simulink library "DAEMOT_Lib"  (R2019b)
settings: Solver=ode45  StartTime=0.0  StopTime=10.0  FixedStep=0.1  RelTol=1e-3
undefined symbols (not defined in the file or in its folder): Controller, CP, Ctrl, Ctrl_Fcn, Elec1, f, F2, Fluid, lag1, Mission, Moody, PropellerProp, rev_comms_sink
libraries: $bdroot x200, instrumentlib x21, simulink x5, dspsigops x2
(part 8 of 13)

== system DAEMOT_Lib/Electrical/Shaft ==
  In1 : Inport
  Bus_Sink_1 : BusCreator  Inputs=1
  Data_Sink : Subsystem  LoadFcn=|  InitFcn=|  mask(Data Sink){}
      LoadFcn=|
      | h      = get_param(gcb,'handle');   % Get block handle                           
      | hblock = get(h);     % Parse out handles structure
      | 
      | str = [hblock.Path(numel(bdroot)+2:end), hblock.Name];
      | str(~ismember(str,['A':'Z' 'a':'z' '0':'9' '_'])) = '';                     
      | set_param([gcb, '/global_data_goto'],'GotoTag',['gdata_',str]);
      |                                
      |                                                                                  
      | clear h hblock str
      InitFcn=|
      | h      = get_param(gcb,'handle');   % Get block handle                           
      | hblock = get(h);     % Parse out handles structure
      | 
      | str = [hblock.Path(numel(bdroot)+2:end), hblock.Name];
      | str(~ismember(str,['A':'Z' 'a':'z' '0':'9' '_'])) = '';                     
      | set_param([gcb, '/global_data_goto'],'GotoTag',['gdata_',str]);
      |                                
      |                                                                                  
      | clear h hblock str
      mask help:
      | Input to this block should be a bus signal with named signals.
      |
      | Bus signals sent to this block will be read by the Data Manager.
      | The Data Manager will handle the global routing of signals.
      |
      | This block should be placed under the mask of components.
      settings: CopyFcn=|
      | h      = get_param(gcb,'handle');   % Get block handle
      | hblock = get(h);     % Parse out handles structure
      | 
      | str = [hblock.Path(numel(bdroot)+2:end), hblock.Name];
      | str(~ismember(str,['A':'Z' 'a':'z' '0':'9' '_'])) = '';
      | set_param([gcb, '/global_data_goto'],'GotoTag',['gdata_',str]);
      | 
      | 
      | clear h hblock str
      settings: NameChangeFcn=|
      | h      = get_param(gcb,'handle');   % Get block handle
      | hblock = get(h);     % Parse out handles structure
      | 
      | str = [hblock.Path(numel(bdroot)+2:end), hblock.Name];
      | str(~ismember(str,['A':'Z' 'a':'z' '0':'9' '_'])) = '';
      | set_param([gcb, '/global_data_goto'],'GotoTag',['gdata_',str]);
      | 
      | 
      | clear h hblock str
      mask Display: text(0.25,0.5,'Data Sink')
  Demux_Out_1 : Demux  Outputs=1
  Integrator2 : Integrator  InitialCondition=w_initial
  Mux_In_1 : Mux  Inputs=1
  Mux_In_2 : Mux  Inputs=1
  Selector1 : Selector  InputPortWidth=1  IndexOptions=Index vector (dialog)  Indices=[1 ]  OutputSizes=1
  Selector2 : Selector  InputPortWidth=1  IndexOptions=Index vector (dialog)  Indices=[1 ]  OutputSizes=1
  Sink1 : Subsystem  LoadFcn=rev_comms_sink();  InitFcn=rev_comms_sink();  mask(Sink){}
      mask help: Used for sending data to the upstream component.
      settings: CopyFcn=rev_comms_sink();  NameChangeFcn=rev_comms_sink();
      mask Display: text(0.25,0.5,'Sink')
  Source1 : Subsystem  mask(Source){}
      mask help: Used for receiving data from the downstream component.
      mask init:
      | n_src = gcb;
      | n_src = str2num(n_src(end));
      | try
      |     rev_comms_source(n_src);
      | catch
      | 
      | end
      mask Display: text(0.25,0.5,'Source')
  b1 : BusCreator  Inputs=2
  current : MATLAB Function  TreatAsAtomicUnit=on
  gb1 : BusSelector  OutputSignals=aspeed,torque
  term1 : Terminator
  Out1 : Outport
  wires:
  [omega] -> Demux_Out_1/1
  Demux_Out_1/1 -> Sink1/1(In1)
  [tau_out] -> current/2(tau_out)
  [tau_in] -> current/1(tau_in)
  [tau_in1] -> Mux_In_1/1
  gb1/2 -> [tau_in1]  "<torque>"
  gb1/1 -> term1/1  "<aspeed>"
  In1/1 -> gb1/1
  Integrator2/1 -> [omega]
  Mux_In_1/1 -> Selector1/1
  current/1(omega_dot) -> Integrator2/1
  Bus_Sink_1/1 -> Data_Sink/1(" ")
  [tau_out1] -> Mux_In_2/1
  Mux_In_2/1 -> Selector2/1
  [tau_out1] -> b1/2  "torque"
  [omega] -> b1/1  "aspeed"
  Source1/1(Out1) -> [tau_out1]
  b1/1 -> Out1/1
  Selector1/1 -> [tau_in]
  Selector2/1 -> [tau_out]
  [omega] -> Bus_Sink_1/1  "Speed [rad_s]"

== system DAEMOT_Lib/Electrical/Speed Source ==
  In1 : Inport
  Constant : Constant  Value=0
  Source1 : Subsystem  mask(Source){}
      mask help: Used for receiving data from the downstream component.
      mask init:
      | n_src = gcb;
      | n_src = str2num(n_src(end));
      | try
      |     rev_comms_source(n_src);
      | catch
      | 
      | end
      mask Display: text(0.25,0.5,'Source')
  Terminator : Terminator
  b1 : BusCreator  Inputs=2
  Out1 : Outport  VectorParamsAs1DForOutWhenUnconnected=off
  wires:
  b1/1 -> Out1/1
  In1/1 -> b1/2  "speed"
  Constant/1 -> b1/1  "torque"
  Source1/1(Out1) -> Terminator/1

== system DAEMOT_Lib/Electrical/Thermal Sink ==
  In1 : Inport
  In2 : Inport  Port=2
  Sink1 : $bdroot/Support Functions/Sink
  Terminator : Terminator
  wires:
  In2/1 -> Sink1/1  "Temp"
  In1/1 -> Terminator/1

== system DAEMOT_Lib/Electrical/Thermal Source ==
  In1 : Inport
  Constant : Constant
  Source1 : $bdroot/Support Functions/Source
  Terminator : Terminator
  b1 : BusCreator  Inputs=2
  Out1 : Outport  VectorParamsAs1DForOutWhenUnconnected=off
  wires:
  Source1/1 -> Terminator/1
  b1/1 -> Out1/1
  In1/1 -> b1/2  "Temp"
  Constant/1 -> b1/1  "Q_kW"

== system DAEMOT_Lib/Electrical/Torque Sink ==
  In1 : Inport
  In2 : Inport  Port=2
  Sink1 : Subsystem  LoadFcn=rev_comms_sink();  InitFcn=rev_comms_sink();  mask(Sink){}
      mask help: Used for sending data to the upstream component.
      settings: CopyFcn=rev_comms_sink();  NameChangeFcn=rev_comms_sink();
      mask Display: text(0.25,0.5,'Sink')
  Terminator : Terminator
  wires:
  In2/1 -> Sink1/1(In1)  "current"
  In1/1 -> Terminator/1

== system DAEMOT_Lib/Electrical/UAV ==
  In1 : Inport
  Bus Creator2 : BusCreator  Inputs=2
  Bus Selector2 : BusSelector  OutputSignals=speed,torque
  Data_Sink : $bdroot/Support Functions/Data_Sink
  Integrator : Integrator  InitialCondition=v_initial
  Property : Subsystem
  Sink1 : $bdroot/Support Functions/Sink
  Terminator1 : Terminator
  speed : MATLAB Function  TreatAsAtomicUnit=on
  wires:
  speed/2(tau) -> [tau]
  speed/1(dv_dt) -> Integrator/1
  [omega] -> speed/2(omega), Property/2(w)
  [tau] -> Bus Creator2/1  "Load Torque"
  Bus Creator2/1 -> Data_Sink/1
  [v] -> Bus Creator2/2  "Vehicle Speed"
  Bus Selector2/2 -> Terminator1/1  "<torque>"
  In1/1 -> Bus Selector2/1
  Bus Selector2/1 -> [omega]  "<speed>"
  [tau] -> Sink1/1
  Integrator/1 -> Property/1(v), speed/1(v), [v]
  Property/1(Props) -> speed/3(props)

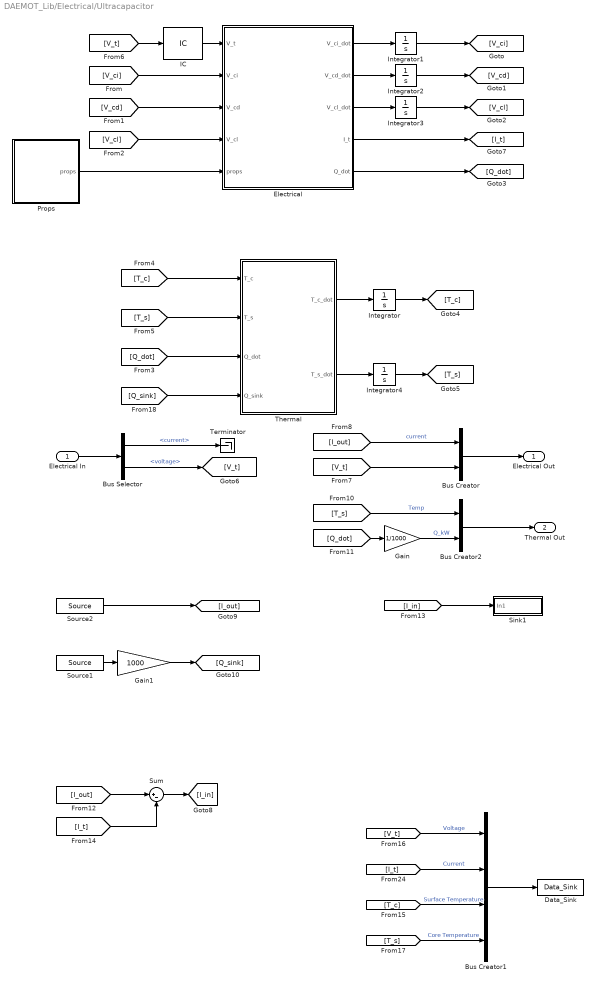
== system DAEMOT_Lib/Electrical/Ultracapacitor ==
  Electrical In : Inport
  Bus Creator : BusCreator  Inputs=2
  Bus Creator1 : BusCreator  Inputs=4
  Bus Creator2 : BusCreator  Inputs=2
  Bus Selector : BusSelector  OutputSignals=current,voltage
  Data_Sink : $bdroot/Support Functions/Data_Sink
  Electrical : MATLAB Function  TreatAsAtomicUnit=on
  Gain : Gain  Gain=1/1000
  Gain1 : Gain  Gain=1000
  IC : InitialCondition  Value=V_0
  Integrator : Integrator  InitialCondition=T_c_0
  Integrator1 : Integrator  InitialCondition=V_0
  Integrator2 : Integrator  InitialCondition=V_0
  Integrator3 : Integrator  InitialCondition=V_0
  Integrator4 : Integrator  InitialCondition=T_s_0
  Props : Subsystem
  Sink1 : Subsystem  LoadFcn=rev_comms_sink();  InitFcn=rev_comms_sink();  mask(Sink){}
      mask help: Used for sending data to the upstream component.
      settings: CopyFcn=rev_comms_sink();  NameChangeFcn=rev_comms_sink();
      mask Display: text(0.25,0.5,'Sink')
  Source1 : $bdroot/Support Functions/Source
  Source2 : $bdroot/Support Functions/Source
  Sum : Sum  Inputs=|+-
  Terminator : Terminator
  Thermal : MATLAB Function  TreatAsAtomicUnit=on
  Electrical Out : Outport  VectorParamsAs1DForOutWhenUnconnected=off
  Thermal Out : Outport  Port=2  VectorParamsAs1DForOutWhenUnconnected=off
  wires:
  [Q_dot] -> Gain/1
  [T_s] -> Bus Creator2/1  "Temp"
  Bus Creator2/1 -> Thermal Out/1
  Integrator4/1 -> [T_s]
  [T_s] -> Thermal/2(T_s)
  [T_c] -> Thermal/1(T_c)
  Integrator/1 -> [T_c]
  Thermal/1(T_c_dot) -> Integrator/1
  Thermal/2(T_s_dot) -> Integrator4/1
  [Q_dot] -> Thermal/3(Q_dot)
  [V_t] -> IC/1
  [V_cl] -> Electrical/4(V_cl)
  [V_cd] -> Electrical/3(V_cd)
  Integrator3/1 -> [V_cl]
  Integrator2/1 -> [V_cd]
  [V_ci] -> Electrical/2(V_ci)
  Integrator1/1 -> [V_ci]
  Electrical/3(V_cl_dot) -> Integrator3/1
  Electrical/2(V_cd_dot) -> Integrator2/1
  Electrical/1(V_ci_dot) -> Integrator1/1
  Electrical In/1 -> Bus Selector/1
  Bus Creator/1 -> Electrical Out/1
  [V_t] -> Bus Creator/2
  [I_out] -> Bus Creator/1  "current"
  Bus Selector/1 -> Terminator/1  "<current>"
  Bus Selector/2 -> [V_t]  "<voltage>"
  [I_in] -> Sink1/1(In1)
  [I_out] -> Sum/1
  [I_t] -> Sum/2
  Sum/1 -> [I_in]
  [T_c] -> Bus Creator1/3  "Surface Temperature"
  [V_t] -> Bus Creator1/1  "Voltage"
  [T_s] -> Bus Creator1/4  "Core Temperature"
  Bus Creator1/1 -> Data_Sink/1
  [I_t] -> Bus Creator1/2  "Current"
  Electrical/4(I_t) -> [I_t]
  IC/1 -> Electrical/1(V_t)
  Source2/1 -> [I_out]
  [Q_sink] -> Thermal/4(Q_sink)
  Gain/1 -> Bus Creator2/2  "Q_kW"
  Source1/1 -> Gain1/1
  Gain1/1 -> [Q_sink]
  Electrical/5(Q_dot) -> [Q_dot]
  Props/1(props) -> Electrical/5(props)

== system DAEMOT_Lib/Electrical/Voltage Bus ==
  In : Inport
  u : Inport  Port=2
  Bus Selector : BusSelector  OutputSignals=current,voltage
  Bus_Sink_1 : BusCreator  Inputs=4
  Data_Sink : $bdroot/Support Functions/Data_Sink
  Demux_Out_1 : Demux  Outputs=2
  Mux_In_1 : Mux  Inputs=2
  Reshape : Reshape
  Selector1 : Selector  InputPortWidth=2  IndexOptions=Index vector (dialog)  Indices=[1 2 ]  OutputSizes=1
  Sink1 : $bdroot/Support Functions/Sink
  Source1 : $bdroot/Support Functions/Source
  Source2 : $bdroot/Support Functions/Source
  Terminator3 : Terminator
  b1 : BusCreator  Inputs=2
  b2 : BusCreator  Inputs=2
  current : MATLAB Function  TreatAsAtomicUnit=on
  voltage : MATLAB Function  TreatAsAtomicUnit=on
  Out1 : Outport  VectorParamsAs1DForOutWhenUnconnected=off
  Out2 : Outport  Port=2  VectorParamsAs1DForOutWhenUnconnected=off
  wires:
  b1/1 -> Out1/1
  In/1 -> Bus Selector/1
  Bus Selector/1 -> Terminator3/1  "<current>"
  Bus Selector/2 -> [V_in]  "<voltage>"
  Source1/1 -> [I_out1]  "I"
  [I_in] -> Sink1/1
  [I_out1] -> b1/1  "current"
  [V_out1] -> b1/2  "voltage"
  voltage/1(V_out) -> Demux_Out_1/1  "voltage"
  Mux_In_1/1 -> Selector1/1
  [I_out1] -> Mux_In_1/1
  current/1(I_in) -> [I_in]
  Bus_Sink_1/1 -> Data_Sink/1
  u/1 -> Reshape/1
  Selector1/1 -> current/1(I_out)
  [V_in] -> voltage/1(V_in)
  Demux_Out_1/1 -> [V_out1]
  [V_out1] -> Bus_Sink_1/1  "voltage1"
  [I_out1] -> Bus_Sink_1/2  "current1"
  [I_out2] -> b2/1  "current"
  [V_out2] -> b2/2  "voltage"
  [V_out2] -> Bus_Sink_1/3  "voltage2"
  [I_out2] -> Bus_Sink_1/4  "current2"
  b2/1 -> Out2/1
  Source2/1 -> [I_out2]
  [I_out2] -> Mux_In_1/2
  Demux_Out_1/2 -> [V_out2]
  Reshape/1 -> current/2(u), voltage/2(u)

== system DAEMOT_Lib/Electrical/Voltage Sink ==
  In1 : Inport
  In2 : Inport  Port=2
  Sink1 : Subsystem  LoadFcn=rev_comms_sink();  InitFcn=rev_comms_sink();  mask(Sink){}
      mask help: Used for sending data to the upstream component.
      settings: CopyFcn=rev_comms_sink();  NameChangeFcn=rev_comms_sink();
      mask Display: text(0.25,0.5,'Sink')
  Terminator : Terminator
  wires:
  In2/1 -> Sink1/1(In1)  "voltage"
  In1/1 -> Terminator/1

== system DAEMOT_Lib/Electrical/Voltage Source ==
  In1 : Inport
  Constant : Constant  Value=0
  Source1 : Subsystem  mask(Source){}
      mask help: Used for receiving data from the downstream component.
      mask init:
      | n_src = gcb;
      | n_src = str2num(n_src(end));
      | try
      |     rev_comms_source(n_src);
      | catch
      | 
      | end
      mask Display: text(0.25,0.5,'Source')
  Terminator : Terminator
  b1 : BusCreator  Inputs=2
  Out1 : Outport  VectorParamsAs1DForOutWhenUnconnected=off
  wires:
  Constant/1 -> b1/1  "current"
  Source1/1(Out1) -> Terminator/1
  In1/1 -> b1/2  "voltage"
  b1/1 -> Out1/1

== system DAEMOT_Lib/Electrical/wye2del ==
  In1 : Inport
  Bus Creator2 : BusCreator  Inputs=2
  Bus Creator3 : BusCreator  Inputs=2
  Bus Selector1 : BusSelector  OutputSignals=current,voltage
  Data_Sink : Subsystem  LoadFcn=|  InitFcn=|  mask(Data Sink){}
      LoadFcn=|
      | h      = get_param(gcb,'handle');   % Get block handle                           
      | hblock = get(h);     % Parse out handles structure
      | 
      | str = [hblock.Path(numel(bdroot)+2:end), hblock.Name];
      | str(~ismember(str,['A':'Z' 'a':'z' '0':'9' '_'])) = '';                     
      | set_param([gcb, '/global_data_goto'],'GotoTag',['gdata_',str]);
      |                                
      |                                                                                  
      | clear h hblock str
      InitFcn=|
      | h      = get_param(gcb,'handle');   % Get block handle                           
      | hblock = get(h);     % Parse out handles structure
      | 
      | str = [hblock.Path(numel(bdroot)+2:end), hblock.Name];
      | str(~ismember(str,['A':'Z' 'a':'z' '0':'9' '_'])) = '';                     
      | set_param([gcb, '/global_data_goto'],'GotoTag',['gdata_',str]);
      |                                
      |                                                                                  
      | clear h hblock str
      mask help:
      | Input to this block should be a bus signal with named signals.
      |
      | Bus signals sent to this block will be read by the Data Manager.
      | The Data Manager will handle the global routing of signals.
      |
      | This block should be placed under the mask of components.
      settings: CopyFcn=|
      | h      = get_param(gcb,'handle');   % Get block handle
      | hblock = get(h);     % Parse out handles structure
      | 
      | str = [hblock.Path(numel(bdroot)+2:end), hblock.Name];
      | str(~ismember(str,['A':'Z' 'a':'z' '0':'9' '_'])) = '';
      | set_param([gcb, '/global_data_goto'],'GotoTag',['gdata_',str]);
      | 
      | 
      | clear h hblock str
      settings: NameChangeFcn=|
      | h      = get_param(gcb,'handle');   % Get block handle
      | hblock = get(h);     % Parse out handles structure
      | 
      | str = [hblock.Path(numel(bdroot)+2:end), hblock.Name];
      | str(~ismember(str,['A':'Z' 'a':'z' '0':'9' '_'])) = '';
      | set_param([gcb, '/global_data_goto'],'GotoTag',['gdata_',str]);
      | 
      | 
      | clear h hblock str
      mask Display: text(0.25,0.5,'Data Sink')
  Gain : Gain  Gain=sqrt(3)
  Gain1 : Gain  Gain=sqrt(3)
  Sink1 : Subsystem  LoadFcn=rev_comms_sink();  InitFcn=rev_comms_sink();  mask(Sink){}
      mask help: Used for sending data to the upstream component.
      settings: CopyFcn=rev_comms_sink();  NameChangeFcn=rev_comms_sink();
      mask Display: text(0.25,0.5,'Sink')
  Source1 : Subsystem  mask(Source){}
      mask help: Used for receiving data from the downstream component.
      mask init:
      | n_src = gcb;
      | n_src = str2num(n_src(end));
      | try
      |     rev_comms_source(n_src);
      | catch
      | 
      | end
      mask Display: text(0.25,0.5,'Source')
  Terminator : Terminator
  Out1 : Outport
  wires:
  [I_in] -> Bus Creator2/1  "Current In [A]"
  [V_out] -> Bus Creator2/2  "Voltage Out [V]"
  Bus Creator2/1 -> Data_Sink/1(" ")
  [I_out] -> Bus Creator3/1  "current"
  Source1/1(Out1) -> [I_out]
  Bus Selector1/1 -> Terminator/1  "<current>"
  Bus Selector1/2 -> [V_in]  "<voltage>"
  [V_out] -> Bus Creator3/2  "voltage"
  [I_in] -> Sink1/1(In1)
  In1/1 -> Bus Selector1/1  "electric"
  Bus Creator3/1 -> Out1/1
  [V_in] -> Gain/1
  Gain/1 -> [V_out]
  [I_out] -> Gain1/1
  Gain1/1 -> [I_in]

== system DAEMOT_Lib/Legacy Components/Aircraft ==
  In1 : Inport
  Aircraft : MATLAB Function  TreatAsAtomicUnit=on
  Bus Creator2 : BusCreator  Inputs=1
  Data_Sink1 : $bdroot/Support Functions/Data_Sink
  Integrate : Integrator  InitialCondition=Vel_init
  Source1 : $bdroot/Support Functions/Source
  Source2 : $bdroot/Support Functions/Source
  b1 : BusCreator  Inputs=2
  b2 : BusCreator  Inputs=2
  Out1 : Outport  VectorParamsAs1DForOutWhenUnconnected=off
  Out2 : Outport  Port=2  VectorParamsAs1DForOutWhenUnconnected=off
  wires:
  In1/1 -> [M_fuel]
  [Vel] -> Bus Creator2/1  "Velocity"
  Bus Creator2/1 -> Data_Sink1/1
  [M_fuel] -> Aircraft/4(M_fuel)
  Integrate/1 -> Aircraft/1(x), [Vel]
  Aircraft/1(x_dot) -> Integrate/1
  [Thrust_2] -> Aircraft/3(Thrust_2)
  [Thrust_1] -> Aircraft/2(Thrust_1)
  b1/1 -> Out1/1
  [Vel] -> b1/1  "Velocity"
  [Thrust_1] -> b1/2  "Thrust"
  b2/1 -> Out2/1
  [Vel] -> b2/1  "Velocity"
  [Thrust_2] -> b2/2  "Thrust"
  Source1/1 -> [Thrust_1]
  Source2/1 -> [Thrust_2]

== system DAEMOT_Lib/Legacy Components/Battery ==
  In1 : Inport
  In2 : Inport  Port=2
  Battery : MATLAB Function  TreatAsAtomicUnit=on
  Bus Selector : BusSelector  OutputSignals=V,I
  Data_Sink1 : $bdroot/Support Functions/Data_Sink
  Integrate : Integrator  InitialCondition=[SOC0]
  P : Constant  Value=P_max
  Product : Product
  Sink1 : $bdroot/Support Functions/Sink
  Source1 : $bdroot/Support Functions/Source
  Terminator3 : Terminator
  b1 : BusCreator  Inputs=3
  b2 : BusCreator  Inputs=2
  eta : Fcn  Expr=a*u^2+b*u+c
  Out1 : Outport  VectorParamsAs1DForOutWhenUnconnected=off
  wires:
  Bus Selector/1 -> [V_in]  "<V>"
  Bus Selector/2 -> Terminator3/1  "<I>"
  [I_in] -> Sink1/1  "I"
  In1/1 -> Bus Selector/1
  P/1 -> Product/1
  In2/1 -> Product/2
  b1/1 -> Data_Sink1/1
  [P] -> b1/2  "Power"
  b2/1 -> Out1/1
  [T] -> b2/1  "T"
  [Q] -> b2/2  "Q_kW"
  Source1/1 -> [T]
  Battery/3(Q) -> [Q]
  Product/1 -> [P]  "Power"
  [Q] -> b1/3  "Q_kW"
  [SOC] -> b1/1  "SOC"
  [T] -> eta/1
  eta/1 -> [eta]
  Battery/1(x_dot) -> Integrate/1
  Integrate/1 -> Battery/1(x), [SOC]
  [eta] -> Battery/4(eta)
  [P] -> Battery/3(P)
  [V_in] -> Battery/2(V_in)
  Battery/2(I_in) -> [I_in]

== system DAEMOT_Lib/Legacy Components/Bus ==
  In : Inport
  Add : Sum
  Bus Creator1 : BusCreator  Inputs=2
  Bus Creator2 : BusCreator  Inputs=2
  Bus Selector : BusSelector  OutputSignals=V,I
  Sink1 : $bdroot/Support Functions/Sink
  Source1 : $bdroot/Support Functions/Source
  Source2 : $bdroot/Support Functions/Source
  Terminator3 : Terminator
  Out1 : Outport  VectorParamsAs1DForOutWhenUnconnected=off
  Out2 : Outport  Port=2  VectorParamsAs1DForOutWhenUnconnected=off
  wires:
  Source1/1 -> Add/1, Bus Creator1/2  "I"
  Bus Selector/2 -> Terminator3/1  "<I>"
  In/1 -> Bus Selector/1
  Bus Creator1/1 -> Out1/1
  Bus Selector/1 -> Bus Creator2/1, Bus Creator1/1  "<V>"
  Bus Creator2/1 -> Out2/1
  Source2/1 -> Add/2, Bus Creator2/2  "I"
  Add/1 -> Sink1/1

== system DAEMOT_Lib/Legacy Components/Bus1 ==
  In : Inport
  Add : Sum  Inputs=2
  Sink1 : $bdroot/Support Functions/Sink
  Source1 : $bdroot/Support Functions/Source
  Source2 : $bdroot/Support Functions/Source
  Terminator3 : Terminator
  b1 : BusCreator  Inputs=2
  b2 : BusCreator  Inputs=2
  in : BusSelector  OutputSignals=V,I
  Out1 : Outport  VectorParamsAs1DForOutWhenUnconnected=off
  Out2 : Outport  Port=2  VectorParamsAs1DForOutWhenUnconnected=off
  wires:
  Source1/1 -> Add/1, b1/2  "I"
  in/2 -> Terminator3/1  "<I>"
  In/1 -> in/1
  b1/1 -> Out1/1
  in/1 -> b1/1, b2/1  "<V>"
  Add/1 -> Sink1/1
  Source2/1 -> b2/2, Add/2  "I"
  b2/1 -> Out2/1

== system DAEMOT_Lib/Legacy Components/Cabin ==
  In1 : Inport
  Heat : Inport  Port=2
  Add1 : Sum
  Add2 : Sum  Inputs=+-
  Bus Creator : BusCreator  Inputs=2
  Bus Creator1 : BusCreator  Inputs=1
  Bus Selector : BusSelector  OutputSignals=mdot_kgps,T_C
  C : Constant  Value=V*Fluid.cp*Fluid.rho
  Divide1 : Product  Inputs=***
  Divide5 : Product  Inputs=*/
  T_cabin : Integrator  InitialCondition=T_init
  cp : Constant  Value=Fluid.cp
  data_sink : $bdroot/Support Functions/Data_Sink
  Out1 : Outport  VectorParamsAs1DForOutWhenUnconnected=off
  wires:
  [T_cabin] -> Add2/2
  [T_in] -> Add2/1
  [m_dot1] -> Divide1/2
  cp/1 -> Divide1/3
  Add2/1 -> Divide1/1
  Divide1/1 -> Add1/2
  [Q_Load1] -> Add1/1
  Add1/1 -> Divide5/1
  C/1 -> Divide5/2
  Heat/1 -> [Q_Load1]
  Divide5/1 -> T_cabin/1
  T_cabin/1 -> [T_cabin]
  Bus Selector/1 -> [m_dot1]  "<mdot_kgps>"
  [T_cabin] -> Bus Creator1/1, Bus Creator/2  "T_C"
  Bus Selector/2 -> [T_in]  "<T_C>"
  [m_dot1] -> Bus Creator/1  "mdot_kgps"
  Bus Creator/1 -> Out1/1
  In1/1 -> Bus Selector/1
  Bus Creator1/1 -> data_sink/1  "Thermal Zone"

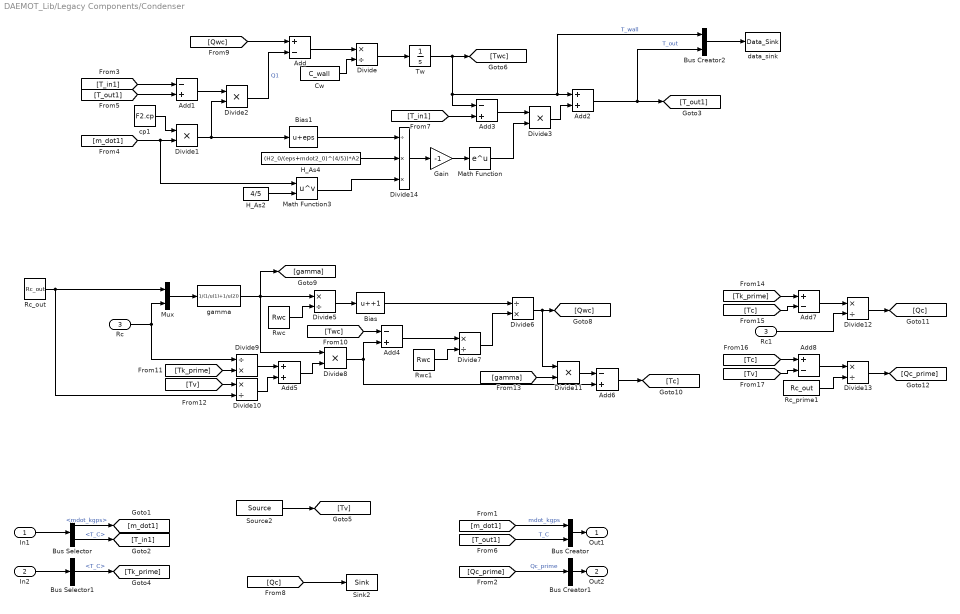
== system DAEMOT_Lib/Legacy Components/Condenser ==
  In1 : Inport
  In2 : Inport  Port=2
  Rc : Inport  Port=3
  Add : Sum  Inputs=+-
  Add{1,3..4,6} (4 alike) : Sum  Inputs=-+
  Add2 : Sum
  Add5 : Sum
  Add7 : Sum  Inputs=+-
  Add8 : Sum  Inputs=+-
  Bias : Bias  Bias=+1
  Bias1 : Bias  Bias=eps
  Bus Creator : BusCreator  Inputs=2
  Bus Creator1 : BusCreator  Inputs=1
  Bus Creator2 : BusCreator  Inputs=2
  Bus Selector : BusSelector  OutputSignals=mdot_kgps,T_C
  Bus Selector1 : BusSelector  OutputSignals=T_C
  Cw : Constant  Value=C_wall
  Divide{,5,7,10,12..13} (6 alike) : Product  Inputs=*/
  Divide{1..3,8,11} (5 alike) : Product  Inputs=**
  Divide14 : Product  Inputs=/**
  Divide6 : Product  Inputs=/*
  Divide9 : Product  Inputs=/*
  Gain : Gain  Gain=-1
  H_As2 : Constant  Value=4/5
  H_As4 : Constant  Value=(H2_0/(eps+mdot2_0)^(4/5))*A2
  Math Function : Math  SaturateOnIntegerOverflow=on
  Math Function3 : Math  Operator=pow  SaturateOnIntegerOverflow=on
  Mux : Mux  Inputs=2
  Rc1 : InportShadow  Port=3
  Rc_out : Constant  Value=Rc_out
  Rc_prime1 : Constant  Value=Rc_out
  Rwc : Constant  Value=Rwc
  Rwc1 : Constant  Value=Rwc
  Sink2 : $bdroot/Support Functions/Sink
  Source2 : $bdroot/Support Functions/Source
  Tw : Integrator  InitialCondition=T_init
  cp1 : Constant  Value=F2.cp
  data_sink : $bdroot/Support Functions/Data_Sink
  gamma : Fcn  Expr=1/(1/u(1)+1/u(2))
  Out1 : Outport  VectorParamsAs1DForOutWhenUnconnected=off
  Out2 : Outport  Port=2  VectorParamsAs1DForOutWhenUnconnected=off
  wires:
  Bias1/1 -> Divide14/1
  Source2/1 -> [Tv]
  Bus Selector/1 -> [m_dot1]  "<mdot_kgps>"
  Bus Creator1/1 -> Out2/1
  Gain/1 -> Math Function/1
  H_As4/1 -> Divide14/2
  Divide14/1 -> Gain/1
  Divide1/1 -> Bias1/1, Divide2/2
  Add1/1 -> Divide2/1
  Math Function/1 -> Divide3/2
  [T_in1] -> Add3/2
  [T_out1] -> Bus Creator/2  "T_C"
  [T_out1] -> Add1/2
  [T_in1] -> Add1/1
  Bus Selector/2 -> [T_in1]  "<T_C>"
  [m_dot1] -> Bus Creator/1  "mdot_kgps"
  Bus Creator/1 -> Out1/1
  Add3/1 -> Divide3/1
  Divide3/1 -> Add2/2
  Divide2/1 -> Add/2  "Q1"
  Add2/1 -> Bus Creator2/2, [T_out1]  "T_out"
  cp1/1 -> Divide1/1
  In1/1 -> Bus Selector/1
  Add/1 -> Divide/1
  Cw/1 -> Divide/2
  Divide/1 -> Tw/1
  Tw/1 -> [Twc], Add3/1, Bus Creator2/1, Add2/1  "T_wall"
  [Qwc] -> Add/1
  [Qc_prime] -> Bus Creator1/1  "Qc_prime"
  [Qc] -> Sink2/1
  In2/1 -> Bus Selector1/1
  Bus Selector1/1 -> [Tk_prime]  "<T_C>"
  Mux/1 -> gamma/1
  Rc/1 -> Divide9/1, Mux/2
  gamma/1 -> [gamma], Divide8/1, Divide5/1
  Rwc/1 -> Divide5/2
  Divide5/1 -> Bias/1
  Bias/1 -> Divide6/1
  Rwc1/1 -> Divide7/2
  Divide7/1 -> Divide6/2
  Add4/1 -> Divide7/1
  [Twc] -> Add4/1
  Divide8/1 -> Add6/2, Add4/2
  Add5/1 -> Divide8/2
  Divide9/1 -> Add5/1
  Divide10/1 -> Add5/2
  [Tk_prime] -> Divide9/2
  [Tv] -> Divide10/1
  Rc_out/1 -> Divide10/2, Mux/1
  Divide6/1 -> Divide11/1, [Qwc]
  Divide11/1 -> Add6/1
  [gamma] -> Divide11/2
  Add6/1 -> [Tc]
  Divide12/1 -> [Qc]
  Rc1/1 -> Divide12/2
  Add7/1 -> Divide12/1
  [Tk_prime] -> Add7/1
  [Tc] -> Add7/2
  Divide13/1 -> [Qc_prime]
  Rc_prime1/1 -> Divide13/2
  Add8/1 -> Divide13/1
  [Tc] -> Add8/1
  [Tv] -> Add8/2
  [m_dot1] -> Math Function3/1, Divide1/2
  Math Function3/1 -> Divide14/3
  H_As2/1 -> Math Function3/2
  Bus Creator2/1 -> data_sink/1

== system DAEMOT_Lib/Legacy Components/Converter ==
  In1 : Inport
  Constant : Constant  Value=V
  Constant1 : Constant  Value=0
  Converter : MATLAB Function  TreatAsAtomicUnit=on
  Data_Sink1 : $bdroot/Support Functions/Data_Sink
  Sink1 : $bdroot/Support Functions/Sink
  Source1 : $bdroot/Support Functions/Source
  Source2 : $bdroot/Support Functions/Source
  Switch : Switch  Criteria=u2 > Threshold
  Terminator2 : Terminator
  b1 : BusCreator  Inputs=5
  b2 : BusCreator  Inputs=2
  b3 : BusCreator  Inputs=2
  gb1 : BusSelector  OutputSignals=V,I
  Out1 : Outport  VectorParamsAs1DForOutWhenUnconnected=off
  Out2 : Outport  Port=2  VectorParamsAs1DForOutWhenUnconnected=off
  wires:
  [I_in] -> Sink1/1
  b1/1 -> Data_Sink1/1
  gb1/1 -> [V_in]  "<V>"
  In1/1 -> gb1/1
  gb1/2 -> Terminator2/1  "<I>"
  Converter/1(I_in) -> [I_in]  "I"
  [I_in] -> b1/1  "Current_in"
  Converter/2(Q) -> [Q]  "Heat Generated [kW]"
  [Q] -> b1/3  "Q_kW"
  b2/1 -> Out1/1
  [V] -> b2/1  "V"
  [I] -> b2/2  "I"
  [I] -> Converter/2(I)
  [V_in] -> Converter/1(V_in)
  Source1/1 -> [I]
  [I] -> b1/2  "Current"
  Constant1/1 -> Switch/3
  Constant/1 -> Switch/1
  Switch/1 -> [V]
  [V_in] -> Switch/2
  Converter/3(eta) -> [eta]  "eta"
  [eta] -> b1/4  "eta"
  Source2/1 -> [T]
  b3/1 -> Out2/1
  [T] -> b3/1  "T"
  [Q] -> b3/2  "Q_kW"
  [T] -> b1/5  "T"

== system DAEMOT_Lib/Legacy Components/Dist ==
  In1 : Inport
  In2 : Inport  Port=2
  u : Inport  Port=3
  Bus Creator1 : BusCreator  Inputs=2
  Bus Selector : BusSelector  OutputSignals=V,I
  Bus Selector1 : BusSelector  OutputSignals=V,I
  Constant : Constant  Value=0
  Demux : Demux  Outputs=2
  MinMax : MinMax
  Mux : Mux  Inputs=2
  Product : Product  Multiplication=Matrix(*)
  Sink1 : $bdroot/Support Functions/Sink
  Sink2 : $bdroot/Support Functions/Sink
  Source1 : $bdroot/Support Functions/Source
  Switch : Switch  Criteria=u2 > Threshold
  Terminator1 : Terminator
  Terminator3 : Terminator
  Out : Outport  VectorParamsAs1DForOutWhenUnconnected=off
  wires:
  [I] -> Bus Creator1/2  "I"
  Bus Selector/2 -> Terminator3/1  "<I>"
  In1/1 -> Bus Selector/1
  Bus Creator1/1 -> Out/1
  Bus Selector/1 -> Mux/1  "<V>"
  Source1/1 -> [I]  "I"
  Bus Selector1/2 -> Terminator1/1  "<I>"
  In2/1 -> Bus Selector1/1
  Bus Selector1/1 -> Mux/2  "<V>"
  MinMax/1 -> Switch/2, [V]  "Voltage"
  Switch/1 -> [I_ins]  "Current"
  [I] -> Product/2
  [V_ins] -> MinMax/1
  Mux/1 -> [V_ins]
  u/1 -> [u]
  [V] -> Bus Creator1/1  "V"
  [I_ins] -> Demux/1
  Demux/2 -> Sink2/1
  Demux/1 -> Sink1/1
  [u] -> Product/1
  Constant/1 -> Switch/3
  Product/1 -> Switch/1  "Current"

== system DAEMOT_Lib/Legacy Components/Dist1 ==
  In1 : Inport
  In2 : Inport  Port=2
  u : Inport  Port=3
  Bus Creator1 : BusCreator  Inputs=2
  Constant : Constant  Value=0
  Demux : Demux  Outputs=2
  MinMax : MinMax
  Mux : Mux  Inputs=2
  Product : Product  Multiplication=Matrix(*)
  Sink1 : $bdroot/Support Functions/Sink
  Sink2 : $bdroot/Support Functions/Sink
  Source1 : $bdroot/Support Functions/Source
  Switch : Switch  Criteria=u2 > Threshold
  b1 : BusSelector  OutputSignals=V,I
  b2 : BusSelector  OutputSignals=V,I
  term1 : Terminator
  term2 : Terminator
  Out : Outport  VectorParamsAs1DForOutWhenUnconnected=off
  wires:
  [I] -> Bus Creator1/2  "I"
  Bus Creator1/1 -> Out/1
  Source1/1 -> [I]  "I"
  MinMax/1 -> Switch/2, [V]  "Voltage"
  Switch/1 -> [I_ins]  "Current"
  [I] -> Product/2
  [V_ins] -> MinMax/1
  Mux/1 -> [V_ins]
  [V] -> Bus Creator1/1  "V"
  [I_ins] -> Demux/1
  [u] -> Product/1
  Constant/1 -> Switch/3
  Product/1 -> Switch/1  "Current"
  In1/1 -> b1/1
  b1/2 -> term1/1  "<I>"
  b1/1 -> Mux/1  "<V>"
  Demux/1 -> Sink1/1
  In2/1 -> b2/1
  b2/1 -> Mux/2  "<V>"
  b2/2 -> term2/1  "<I>"
  Demux/2 -> Sink2/1
  u/1 -> [u]

== system DAEMOT_Lib/Legacy Components/Engine ==
  In1 : Inport
  In2 : Inport  Port=2
  Constant : Constant  Value=P
  Constant1 : Constant  Value=Fuel.U
  Data_Sink1 : $bdroot/Support Functions/Data_Sink
  Engine : MATLAB Function  TreatAsAtomicUnit=on
  Integrate : Integrator  InitialCondition=[Omega_init]
  Sink1 : $bdroot/Support Functions/Sink
  Sink2 : $bdroot/Support Functions/Sink
  Source1 : $bdroot/Support Functions/Source
  Source2 : $bdroot/Support Functions/Source
  Terminator1 : Terminator
  Terminator3 : Terminator
  Terminator4 : Terminator
  b1 : BusCreator  Inputs=4
  b2 : BusCreator  Inputs=2
  b3 : BusCreator  Inputs=2
  gb1 : BusSelector  OutputSignals=Velocity,Thrust
  gb2 : BusSelector  OutputSignals=mdot_kgps,T_C,P_kPa
  Out1 : Outport  VectorParamsAs1DForOutWhenUnconnected=off
  Out2 : Outport  Port=2  VectorParamsAs1DForOutWhenUnconnected=off
  wires:
  [T] -> b1/4  "T"
  [Q] -> b3/2  "Q_kW"
  [T] -> b3/1  "T"
  b3/1 -> Out2/1
  Source2/1 -> [T]
  [Thrust] -> Sink1/1
  In1/1 -> gb1/1
  gb1/1 -> [Vel]  "<Velocity>"
  gb1/2 -> Terminator3/1  "<Thrust>"
  Source1/1 -> [Torque]
  [Omega] -> b2/2  "Omega"
  [Torque] -> b2/1  "Torque"
  b2/1 -> Out1/1
  [Q] -> b1/3  "Q"
  Engine/3(Q_bearings) -> [Q]  "Heat Generated [kW]"
  [Thrust] -> b1/2  "Thrust"
  Constant1/1 -> Engine/5(U)
  [Torque] -> Engine/4(Torque)
  [Vel] -> Engine/3(Vel)
  [Mdot] -> Engine/2(Mdot)
  Integrate/1 -> Engine/1(x), [Omega]
  Engine/2(Thrust) -> [Thrust]  "Thrust [N]"
  Engine/1(x_dot) -> Integrate/1
  Constant/1 -> [P_out]
  [Omega] -> b1/1  "Omega"
  b1/1 -> Data_Sink1/1
  [P_out] -> Sink2/1
  gb2/3 -> Terminator1/1  "<P_kPa>"
  In2/1 -> gb2/1
  gb2/1 -> [Mdot]  "<mdot_kgps>"
  gb2/2 -> Terminator4/1  "<T_C>"

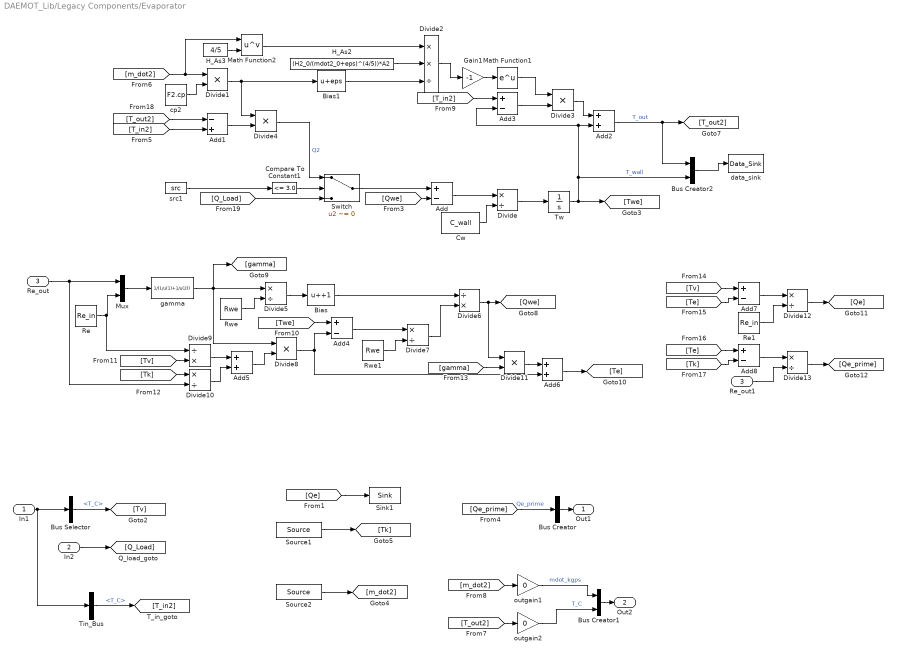
== system DAEMOT_Lib/Legacy Components/Evaporator ==
  In1 : Inport
  In2 : Inport  Port=2
  Re_out : Inport  Port=3
  Add{,3..4,7..8} (5 alike) : Sum  Inputs=+-
  Add1 : Sum  Inputs=-+
  Add2 : Sum
  Add5 : Sum
  Add6 : Sum
  Bias : Bias  Bias=+1
  Bias1 : Bias  Bias=eps
  Bus Creator : BusCreator  Inputs=1
  Bus Creator1 : BusCreator  Inputs=2
  Bus Creator2 : BusCreator  Inputs=2
  Bus Selector : BusSelector  OutputSignals=T_C
  Compare To Constant1 : simulink/Logic and Bit Operations/Compare To Constant  relop=<=  const=3.0  OutDataTypeStr=boolean
  Cw : Constant  Value=C_wall
  Divide{,5,7,10,12..13} (6 alike) : Product  Inputs=*/
  Divide{1,3..4,8,11} (5 alike) : Product  Inputs=**
  Divide2 : Product  Inputs=**/
  Divide6 : Product  Inputs=/*
  Divide9 : Product  Inputs=/*
  Gain1 : Gain  Gain=-1
  H_As2 : Constant  Value=(H2_0/(mdot2_0+eps)^(4/5))*A2
  H_As3 : Constant  Value=4/5
  Math Function1 : Math  SaturateOnIntegerOverflow=on
  Math Function2 : Math  Operator=pow  SaturateOnIntegerOverflow=on
  Mux : Mux  Inputs=2
  Re : Constant  Value=Re_in
  Re1 : Constant  Value=Re_in
  Re_out1 : InportShadow  Port=3
  Rwe : Constant  Value=Rwe
  Rwe1 : Constant  Value=Rwe
  Sink1 : $bdroot/Support Functions/Sink
  Source1 : $bdroot/Support Functions/Source
  Source2 : $bdroot/Support Functions/Source
  Switch : Switch  Criteria=u2 ~= 0
  Tin_Bus : BusSelector  OutputSignals=T_C
  Tw : Integrator  InitialCondition=T_init
  cp2 : Constant  Value=F2.cp
  data_sink : $bdroot/Support Functions/Data_Sink
  gamma : Fcn  Expr=1/(1/u(1)+1/u(2))
  outgain1 : Gain  Gain=0
  outgain2 : Gain  Gain=0
  src1 : Constant  Value=src
  Out1 : Outport  VectorParamsAs1DForOutWhenUnconnected=off
  Out2 : Outport  Port=2  VectorParamsAs1DForOutWhenUnconnected=off
  wires:
  Switch/1 -> Add/1
  [Qwe] -> Add/2
  Divide/1 -> Tw/1
  Cw/1 -> Divide/2
  Add/1 -> Divide/1
  Bus Creator/1 -> Out1/1
  [Qe] -> Sink1/1
  Bus Selector/1 -> [Tv]  "<T_C>"
  Source1/1 -> [Tk]
  [Qe_prime] -> Bus Creator/1  "Qe_prime"
  Mux/1 -> gamma/1
  Re/1 -> Mux/2, Divide9/1
  gamma/1 -> Divide5/1, Divide8/1, [gamma]
  Rwe/1 -> Divide5/2
  Divide5/1 -> Bias/1
  Bias/1 -> Divide6/1
  Rwe1/1 -> Divide7/2
  Divide7/1 -> Divide6/2
  Add4/1 -> Divide7/1
  [Twe] -> Add4/1
  Divide8/1 -> Add4/2, Add6/2
  Add5/1 -> Divide8/2
  Divide9/1 -> Add5/1
  Divide10/1 -> Add5/2
  [Tv] -> Divide9/2
  [Tk] -> Divide10/1
  Re_out/1 -> Mux/1, Divide10/2
  Divide6/1 -> [Qwe], Divide11/1
  Divide11/1 -> Add6/1
  [gamma] -> Divide11/2
  Add6/1 -> [Te]
  Divide12/1 -> [Qe]
  Add7/1 -> Divide12/1
  [Tv] -> Add7/1
  [Te] -> Add7/2
  Divide13/1 -> [Qe_prime]
  Re_out1/1 -> Divide13/2
  Add8/1 -> Divide13/1
  [Te] -> Add8/1
  [Tk] -> Add8/2
  Re1/1 -> Divide12/2
  [T_out2] -> outgain2/1
  [m_dot2] -> outgain1/1
  Source2/1 -> [m_dot2]
  Bias1/1 -> Divide2/3
  [T_in2] -> Add3/1
  Add3/1 -> Divide3/2
  Divide3/1 -> Add2/1
  Add2/1 -> Bus Creator2/1, [T_out2]  "T_out"
  Math Function1/1 -> Divide3/1
  Gain1/1 -> Math Function1/1
  Divide2/1 -> Gain1/1
  H_As2/1 -> Divide2/2
  cp2/1 -> Divide1/2
  Divide1/1 -> Divide4/1, Bias1/1
  [T_out2] -> Add1/1
  [T_in2] -> Add1/2
  Add1/1 -> Divide4/2
  Divide4/1 -> Switch/1  "Q2"
  Tw/1 -> [Twe], Bus Creator2/2, Add2/2, Add3/2  "T_wall"
  [Q_Load] -> Switch/3
  [m_dot2] -> Math Function2/1, Divide1/1
  Math Function2/1 -> Divide2/1
  H_As3/1 -> Math Function2/2
  In1/1 -> Bus Selector/1, Tin_Bus/1
  src1/1 -> Compare To Constant1/1
  Compare To Constant1/1 -> Switch/2
  Bus Creator1/1 -> Out2/1
  Tin_Bus/1 -> [T_in2]  "<T_C>"
  outgain1/1 -> Bus Creator1/1  "mdot_kgps"
  outgain2/1 -> Bus Creator1/2  "T_C"
  In2/1 -> [Q_Load]
  Bus Creator2/1 -> data_sink/1

== system DAEMOT_Lib/Legacy Components/Fan ==
  In1 : Inport
  In2 : Inport  Port=2
  In3 : Inport  Port=3
  Bus Creator2 : BusCreator  Inputs=7
  Constant1 : Constant  Value=T_init
  Constant11 : Constant  Value=T_init
  Constant2 : Constant  Value=P_init
  Constant7 : Constant  Value=P_init
  Data_Sink1 : $bdroot/Support Functions/Data_Sink
  Demux : Demux  Outputs=2
  Integrate : Integrator  InitialCondition=[T_init P_init]
  Pump : MATLAB Function  TreatAsAtomicUnit=on
  Sink1 : $bdroot/Support Functions/Sink
  Sink2 : $bdroot/Support Functions/Sink
  Source1 : $bdroot/Support Functions/Source
  Terminator1 : Terminator
  Terminator2 : Terminator
  b1 : BusCreator  Inputs=3
  gb1 : BusSelector  OutputSignals=mdot_kgps,T_C,P_kPa
  gb2 : BusSelector  OutputSignals=V,I
  n-D Lookup Table1 : Lookup_n-D  BreakpointsForDimension1=Fluid.P  BreakpointsForDimension2=Fluid.T  BreakpointsForDimension3=[5, 7]  Table=Fluid.Rho_pt  ExtrapMethod=Clip  UseLastTableValue=on  RndMeth=Simplest  InputSameDT=on
  n-D Lookup Table2 : Lookup_n-D  BreakpointsForDimension1=Fluid.P  BreakpointsForDimension2=Fluid.T  BreakpointsForDimension3=[5, 7]  Table=Fluid.C_pt  ExtrapMethod=Clip  UseLastTableValue=on  RndMeth=Simplest  InputSameDT=on
  Out1 : Outport  VectorParamsAs1DForOutWhenUnconnected=off
  wires:
  b1/1 -> Out1/1
  [Mdot_down] -> b1/1  "mdot_kgps"
  gb1/2 -> [T_in]  "<T_C>"
  [T_out] -> b1/2  "T_C"
  gb1/1 -> Terminator1/1  "<mdot_kgps>"
  In1/1 -> gb1/1
  [P_out] -> b1/3  "P_kPa"
  gb1/3 -> [P_in]  "<P_kPa>"
  [Mdot] -> Sink1/1
  Source1/1 -> [Mdot_down]
  In3/1 -> [Omega]
  [Omega] -> Pump/6(Omega)
  Pump/3(I) -> [I]
  Bus Creator2/1 -> Data_Sink1/1
  [T_out] -> Bus Creator2/1  "T_out"
  [Mdot] -> Bus Creator2/2  "Mdot"
  [I] -> Bus Creator2/4  "Current"
  [P_in] -> Pump/2(P_in)
  [Mdot_down] -> Pump/5(Mdot_down)
  Integrate/1 -> Demux/1, Pump/1(x)
  Pump/1(x_dot) -> Integrate/1
  [T_in] -> Pump/3(T_in)
  [P_out] -> Bus Creator2/3  "P_out"
  Pump/2(Mdot) -> [Mdot]
  Demux/2 -> [P_out]
  Demux/1 -> [T_out]
  gb2/1 -> [V_in]  "<V>"
  In2/1 -> gb2/1
  gb2/2 -> Terminator2/1  "<I>"
  [I] -> Sink2/1
  [Omega] -> Bus Creator2/5  "Speed"
  [Q] -> Bus Creator2/6  "Q"
  Pump/4(Q) -> [Q]
  [V_in] -> Pump/4(V_in)
  Pump/5(eta) -> [eta]
  [eta] -> Bus Creator2/7  "eta"
  Constant7/1 -> n-D Lookup Table2/1
  Constant11/1 -> n-D Lookup Table2/2
  Constant2/1 -> n-D Lookup Table1/1
  Constant1/1 -> n-D Lookup Table1/2
  n-D Lookup Table1/1 -> Pump/8(rho)
  n-D Lookup Table2/1 -> Pump/7(cp)

== system DAEMOT_Lib/Legacy Components/Fan1 ==
  Flow In : Inport
  ω : Inport  Port=2
  Add1 : Sum  Inputs=-+
  Add4 : Sum
  Add5 : Sum  Inputs=+++
  Bus Creator : BusCreator  Inputs=2
  Bus Creator1 : BusCreator  Inputs=2
  Bus Selector : BusSelector  OutputSignals=T_C
  Bus Selector1 : BusSelector  OutputSignals=mdot_kgps
  Divide1 : Product  Inputs=**
  Divide5 : Product  Inputs=**
  Divide6 : Product  Inputs=**
  Gain : Gain  Gain=1/(tau+eps)
  K : Constant  Value=k
  Math Function1 : Math  Operator=square  SaturateOnIntegerOverflow=on
  Sink1 : Subsystem
      settings: CopyFcn=rev_comms_sink()  NameChangeFcn=rev_comms_sink()
      mask Display: text(0.25,0.5,'Sink')
  Tout : Integrator  InitialCondition=T_init
  alpha : Constant  Value=alpha
  beta : Constant  Value=beta
  data_sink : $bdroot/Support Functions/Data_Sink
  gamma : Constant  Value=gamma
  lambda : Constant  Value=lambda
  Flow Out : Outport  VectorParamsAs1DForOutWhenUnconnected=off
  wires:
  Bus Selector1/1 -> Sink1/1(In1)  "<mdot_kgps>"
  Bus Creator/1 -> Bus Selector1/1, Bus Creator1/2, Flow Out/1  "Flow Out"
  [T_in] -> Add1/2
  Add1/1 -> Gain/1
  Gain/1 -> Tout/1
  Tout/1 -> [T_out], Add1/1
  [T_out] -> Bus Creator/2  "T_C"
  Bus Selector/1 -> [T_in]  "<T_C>"
  alpha/1 -> Divide1/1
  Flow In/1 -> Bus Selector/1
  ω/1 -> Divide1/2, Math Function1/1, Divide6/1
  Divide1/1 -> Add4/1
  beta/1 -> Add4/2
  Add4/1 -> [m_dot]
  Divide5/1 -> Add5/1
  Add5/1 -> Bus Creator1/1  "Power_W"
  K/1 -> Add5/3
  Divide6/1 -> Add5/2
  gamma/1 -> Divide6/2
  lambda/1 -> Divide5/1
  Math Function1/1 -> Divide5/2
  [m_dot] -> Bus Creator/1  "mdot_kgps"
  Bus Creator1/1 -> data_sink/1

== system DAEMOT_Lib/Legacy Components/Flow Flow Source (Pressure) ==
  In2 : Inport
  In3 : Inport  Port=2
  Constant4 : Constant  Value=-1
  Source1 : Subsystem  mask(Source){}
      mask help: Used for receiving data from the downstream component.
      mask init:
      | n_src = gcb;
      | n_src = str2num(n_src(end));
      | try
      |     rev_comms_source(n_src);
      | catch
      | 
      | end
      mask Display: text(0.25,0.5,'Source')
  Terminator : Terminator
  b1 : BusCreator  Inputs=3
  Out1 : Outport  VectorParamsAs1DForOutWhenUnconnected=off
  wires:
  b1/1 -> Out1/1
  Constant4/1 -> b1/1  "mdot_kgps"
  In2/1 -> b1/2  "T_C"
  In3/1 -> b1/3  "P_kPa"
  Source1/1(Out1) -> Terminator/1

== system DAEMOT_Lib/Legacy Components/Flow Sink (Mass Flow Rate) ==
  In4 : Inport
  In3 : Inport  Port=2
  Sink1 : $bdroot/Support Functions/Sink
  Terminator : Terminator
  wires:
  In3/1 -> Sink1/1  "mdot_kgps"
  In4/1 -> Terminator/1

== system DAEMOT_Lib/Legacy Components/Flow Sink (Pressure) ==
  In4 : Inport
  In3 : Inport  Port=2
  Sink1 : $bdroot/Support Functions/Sink
  Terminator : Terminator
  wires:
  In3/1 -> Sink1/1  "P_kPa"
  In4/1 -> Terminator/1

== system DAEMOT_Lib/Legacy Components/Flow Source (Mass Flow Rate) ==
  In1 : Inport
  In2 : Inport  Port=2
  Constant4 : Constant  Value=-1
  Source1 : Subsystem  mask(Source){}
      mask help: Used for receiving data from the downstream component.
      mask init:
      | n_src = gcb;
      | n_src = str2num(n_src(end));
      | try
      |     rev_comms_source(n_src);
      | catch
      | 
      | end
      mask Display: text(0.25,0.5,'Source')
  Terminator : Terminator
  b1 : BusCreator  Inputs=3
  Out1 : Outport  VectorParamsAs1DForOutWhenUnconnected=off
  wires:
  b1/1 -> Out1/1
  In1/1 -> b1/2  "T_C"
  In2/1 -> b1/1  "mdot_kgps"
  Constant4/1 -> b1/3  "P_kPa"
  Source1/1(Out1) -> Terminator/1

== system DAEMOT_Lib/Legacy Components/Flow Split_Junction_Wall ==
  In1 : Inport
  In2 : Inport  Port=2
  Bus Creator2 : BusCreator  Inputs=3
  Constant5 : Constant  Value=Fluid.Bulk_Mod
  Demux : Demux  Outputs=3
  Dynamic_Flow_Split_Junction : MATLAB Function  TreatAsAtomicUnit=on
  Integrator1 : Integrator  InitialCondition=[T_init P_init Tw_init]
  Mux_In_1 : Mux  Inputs=1
  Mux_In_2 : Mux  Inputs=1
  Mux_In_3 : Mux  Inputs=1
  Q_BUS : BusSelector  OutputSignals=Q_kW
  Selector1 : Selector  InputPortWidth=1  IndexOptions=Index vector (dialog)  Indices=[1 ]  OutputSizes=1
  Selector2 : Selector  InputPortWidth=1  IndexOptions=Index vector (dialog)  Indices=[1 ]  OutputSizes=1
  Sink1 : $bdroot/Support Functions/Sink
  Source1 : Subsystem
      mask init:
      | n_src = gcb;
      | n_src = str2num(n_src(end));
      | 
      | rev_comms_source(n_src);
      mask Display: text(0.25,0.5,'Source')
  b1 : BusCreator  Inputs=3
  data_sink1 : $bdroot/Support Functions/Data_Sink
  gb1 : BusSelector  OutputSignals=mdot_kgps,T_C,P_kPa
  gp1 : Terminator
  n-D Lookup Table1 : Lookup_n-D  BreakpointsForDimension1=Fluid.P  BreakpointsForDimension2=Fluid.T  BreakpointsForDimension3=[5, 7]  Table=Fluid.C_pt  ExtrapMethod=Clip  UseLastTableValue=on  RndMeth=Simplest  InputSameDT=on
  n-D Lookup Table2 : Lookup_n-D  BreakpointsForDimension1=Fluid.P  BreakpointsForDimension2=Fluid.T  BreakpointsForDimension3=[5, 7]  Table=Fluid.Rho_pt  ExtrapMethod=Clip  UseLastTableValue=on  RndMeth=Simplest  InputSameDT=on
  n-D Lookup Table3 : Lookup_n-D  BreakpointsForDimension1=Fluid.P  BreakpointsForDimension2=Fluid.T  BreakpointsForDimension3=[5, 7]  Table=Fluid.Rho_pt  ExtrapMethod=Clip  UseLastTableValue=on  RndMeth=Simplest  InputSameDT=on
  n-D Lookup Table8 : Lookup_n-D  BreakpointsForDimension1=Fluid.P  BreakpointsForDimension2=Fluid.T  BreakpointsForDimension3=[5, 7]  Table=Fluid.K_pt  ExtrapMethod=Clip  UseLastTableValue=on  RndMeth=Simplest  InputSameDT=on
  n-D Lookup Table9 : Lookup_n-D  BreakpointsForDimension1=Fluid.P  BreakpointsForDimension2=Fluid.T  BreakpointsForDimension3=[5, 7]  Table=Fluid.Mu_pt  ExtrapMethod=Clip  UseLastTableValue=on  RndMeth=Simplest  InputSameDT=on
  Out1 : Outport  VectorParamsAs1DForOutWhenUnconnected=off
  wires:
  Selector2/1 -> Dynamic_Flow_Split_Junction/4(T_in)
  Demux/2 -> [P]
  Demux/1 -> [T]
  [T] -> n-D Lookup Table2/2
  [P] -> n-D Lookup Table2/1
  n-D Lookup Table2/1 -> Dynamic_Flow_Split_Junction/5(rho)
  Constant5/1 -> Dynamic_Flow_Split_Junction/6(E_fluid)
  Selector1/1 -> Dynamic_Flow_Split_Junction/2(Mdot_in)
  Integrator1/1 -> Demux/1, Dynamic_Flow_Split_Junction/1(x)
  [P] -> Bus Creator2/2  "P"
  [T] -> Bus Creator2/1  "T_out"
  Bus Creator2/1 -> data_sink1/1
  Dynamic_Flow_Split_Junction/1(x_dot) -> Integrator1/1
  [P] -> Sink1/1
  [T_in1] -> Mux_In_3/1
  [M_out1] -> Mux_In_2/1
  [M_in1] -> Mux_In_1/1
  Mux_In_2/1 -> Dynamic_Flow_Split_Junction/3(Mdot_out)
  Mux_In_1/1 -> Selector1/1
  Mux_In_3/1 -> Selector2/1
  gb1/3 -> gp1/1  "<P_kPa>"
  [P] -> b1/3  "P_kPa"
  In1/1 -> gb1/1
  Source1/1(Out1) -> [M_out1]
  gb1/1 -> [M_in1]  "<mdot_kgps>"
  [T] -> b1/2  "T_C"
  gb1/2 -> [T_in1]  "<T_C>"
  [M_out1] -> b1/1  "mdot_kgps"
  b1/1 -> Out1/1
  Q_BUS/1 -> Dynamic_Flow_Split_Junction/7(Q_load)  "<Q_kW>"
  [T_wall] -> Bus Creator2/3  "T_wall"
  Demux/3 -> [T_wall]
  [T] -> n-D Lookup Table3/2, n-D Lookup Table9/2, n-D Lookup Table1/2, n-D Lookup Table8/2
  n-D Lookup Table3/1 -> Dynamic_Flow_Split_Junction/11(Rho)
  [P] -> n-D Lookup Table3/1, n-D Lookup Table1/1, n-D Lookup Table8/1, n-D Lookup Table9/1
  n-D Lookup Table8/1 -> Dynamic_Flow_Split_Junction/9(k)
  n-D Lookup Table9/1 -> Dynamic_Flow_Split_Junction/8(mu)
  n-D Lookup Table1/1 -> Dynamic_Flow_Split_Junction/10(Cp)
  In2/1 -> Q_BUS/1

== system DAEMOT_Lib/Legacy Components/Fluid Tank ==
  In1 : Inport
  In2 : Inport  Port=2
  Bus Creator2 : BusCreator  Inputs=4
  Demux : Demux  Outputs=2
  Integrate : Integrator  InitialCondition=[T_init P_init]
  Sink1 : $bdroot/Support Functions/Sink
  Source1 : $bdroot/Support Functions/Source
  Tank : MATLAB Function  TreatAsAtomicUnit=on
  Terminator : Terminator
  b1 : BusCreator  Inputs=3
  data_sink1 : $bdroot/Support Functions/Data_Sink
  gb1 : BusSelector  OutputSignals=mdot_kgps,T_C,P_kPa
  n-D Lookup Table1 : Lookup_n-D  BreakpointsForDimension1=Fluid.P  BreakpointsForDimension2=Fluid.T  BreakpointsForDimension3=[5, 7]  Table=Fluid.C_pt  ExtrapMethod=Clip  UseLastTableValue=on  RndMeth=Simplest  InputSameDT=on
  n-D Lookup Table2 : Lookup_n-D  BreakpointsForDimension1=Fluid.P  BreakpointsForDimension2=Fluid.T  BreakpointsForDimension3=[5, 7]  Table=Fluid.Rho_pt  ExtrapMethod=Clip  UseLastTableValue=on  RndMeth=Simplest  InputSameDT=on
  Out1 : Outport  VectorParamsAs1DForOutWhenUnconnected=off
  wires:
  b1/1 -> Out1/1
  [Mdot_out] -> b1/1  "mdot_kgps"
  gb1/2 -> [T_in]  "<T_C>"
  [T_tank] -> b1/2  "T_C"
  gb1/1 -> [Mdot_in]  "<mdot_kgps>"
  In1/1 -> gb1/1
  [P_tank] -> b1/3  "P_kPa"
  gb1/3 -> Terminator/1  "<P_kPa>"
  [P_tank] -> Sink1/1
  Source1/1 -> [Mdot_out]
  In2/1 -> [T_amb]
  [Mdot_in] -> Tank/2(Mdot_in)
  [Mdot_out] -> Tank/3(Mdot_out)
  Tank/1(x_dot) -> Integrate/1
  Integrate/1 -> Demux/1, Tank/1(x)
  Demux/1 -> [T_tank]
  Demux/2 -> [P_tank]
  Tank/3(h) -> [h_tank]
  [T_tank] -> n-D Lookup Table2/2, n-D Lookup Table1/2
  [P_tank] -> n-D Lookup Table2/1, n-D Lookup Table1/1
  n-D Lookup Table1/1 -> Tank/6(Cp)
  Tank/2(M) -> [M_tank]
  n-D Lookup Table2/1 -> Tank/7(Rho)
  [T_in] -> Tank/4(T_in)
  [T_amb] -> Tank/5(T_amb)
  Bus Creator2/1 -> data_sink1/1
  [T_tank] -> Bus Creator2/1  "T_tank"
  [P_tank] -> Bus Creator2/2  "P_tank"
  [h_tank] -> Bus Creator2/4  "h_tank"
  [M_tank] -> Bus Creator2/3  "M_tank"

== system DAEMOT_Lib/Legacy Components/From LabVIEW_Old ==
  UDP Receive : instrumentlib/UDP Receive  Host=localhost  Port=61556  LocalPort=61557  EnablePortSharing=off  GetLatestData=off  DataSize=[46 1]  DataType=double  ASCIIFormatting=%f,  Terminator=LF  ByteOrder=BigEndian  EnableBlockingMode=on  Timeout=10  SampleTime=0.1  LocalAddress=0.0.0.0
      settings: SourceProductName=Instrument Control Toolbox
  Out : Outport  VectorParamsAs1DForOutWhenUnconnected=off
  wires:
  UDP Receive/1 -> Out/1

== system DAEMOT_Lib/Legacy Components/Generator ==
  In1 : Inport
  Constant : Constant  Value=V
  Data_Sink1 : $bdroot/Support Functions/Data_Sink
  Generator : MATLAB Function  TreatAsAtomicUnit=on
  Sink1 : $bdroot/Support Functions/Sink
  Source1 : $bdroot/Support Functions/Source
  Source2 : $bdroot/Support Functions/Source
  Terminator2 : Terminator
  b1 : BusCreator  Inputs=4
  b2 : BusCreator  Inputs=2
  b3 : BusCreator  Inputs=2
  gb1 : BusSelector  OutputSignals=Torque,Omega
  Out1 : Outport  VectorParamsAs1DForOutWhenUnconnected=off
  Out2 : Outport  Port=2  VectorParamsAs1DForOutWhenUnconnected=off
  wires:
  [Torque] -> Sink1/1
  b1/1 -> Data_Sink1/1
  gb1/1 -> Terminator2/1  "<Torque>"
  In1/1 -> gb1/1
  gb1/2 -> [Omega]  "<Omega>"
  Constant/1 -> [V]
  Generator/1(Torque) -> [Torque]  "Torque [Nm]"
  [Torque] -> b1/1  "Torque"
  Generator/2(Q) -> [Q]  "Heat Generated [kW]"
  [Q] -> b1/3  "Q_kW"
  b2/1 -> Out1/1
  [V] -> b2/1  "V"
  [I] -> b2/2  "I"
  [I] -> Generator/2(I)
  [Omega] -> Generator/1(Omega)
  Source1/1 -> [I]
  [I] -> b1/2  "Current"
  Source2/1 -> [T]
  b3/1 -> Out2/1
  [T] -> b3/1  "T"
  [Q] -> b3/2  "Q_kW"
  [T] -> b1/4  "T"

== system DAEMOT_Lib/Legacy Components/Graph Sink ==
  In1 : Inport
  Sink1 : Subsystem  LoadFcn=rev_comms_sink();  InitFcn=rev_comms_sink();  mask(Sink){}
      mask help: Used for sending data to the upstream component.
      settings: CopyFcn=rev_comms_sink();  NameChangeFcn=rev_comms_sink();
      mask Display: text(0.25,0.5,'Sink')
  Terminator : Terminator
  val : Constant  Value=value
  wires:
  val/1 -> Sink1/1(In1)
  In1/1 -> Terminator/1

== system DAEMOT_Lib/Legacy Components/Graph Source ==
  Constant : Constant  Value=0
  Source1 : Subsystem  mask(Source){}
      mask help: Used for receiving data from the downstream component.
      mask init:
      | n_src = gcb;
      | n_src = str2num(n_src(end));
      | try
      |     rev_comms_source(n_src);
      | catch
      | 
      | end
      mask Display: text(0.25,0.5,'Source')
  Terminator : Terminator
  b1 : BusCreator  Inputs=2
  val : Constant  Value=value
  Out1 : Outport  VectorParamsAs1DForOutWhenUnconnected=off
  wires:
  val/1 -> b1/2  "voltage"
  Constant/1 -> b1/1  "current"
  Source1/1(Out1) -> Terminator/1
  b1/1 -> Out1/1

== system DAEMOT_Lib/Legacy Components/Heat Sink (Temp) ==
  In1 : Inport
  In2 : Inport  Port=2
  Sink1 : Subsystem  LoadFcn=rev_comms_sink();  InitFcn=rev_comms_sink();  mask(Sink){}
      mask help: Used for sending data to the upstream component.
      settings: CopyFcn=rev_comms_sink();  NameChangeFcn=rev_comms_sink();
      mask Display: text(0.25,0.5,'Sink')
  Terminator : Terminator
  wires:
  In1/1 -> Terminator/1
  In2/1 -> Sink1/1(In1)  "T"

== system DAEMOT_Lib/Legacy Components/Heater ==
  In1 : Inport
  In2 : Inport  Port=2
  Bus Selector : BusSelector  OutputSignals=V,I
  Constant : Constant  Value=0
  Constant1 : Constant  Value=0
  Data_Sink1 : $bdroot/Support Functions/Data_Sink
  Divide : Product  Inputs=/
  Gain : Gain  Gain=1000
  P : Constant  Value=P_max
  Product : Product
  Product1 : Product
  Sink1 : $bdroot/Support Functions/Sink
  Source1 : $bdroot/Support Functions/Source
  Switch : Switch  Criteria=u2 > Threshold
  Switch1 : Switch  Criteria=u2 > Threshold
  Terminator3 : Terminator
  b1 : BusCreator  Inputs=2
  b2 : BusCreator  Inputs=2
  Out1 : Outport  VectorParamsAs1DForOutWhenUnconnected=off
  wires:
  Bus Selector/1 -> Divide/1, Switch/2, Switch1/2  "<V>"
  Bus Selector/2 -> Terminator3/1  "<I>"
  Product1/1 -> Gain/1  "I"
  In1/1 -> Bus Selector/1
  P/1 -> Product/1
  In2/1 -> Product/2
  Switch/1 -> Product1/1
  Divide/1 -> Switch/1
  Constant/1 -> Switch/3
  b1/1 -> Data_Sink1/1
  Switch1/1 -> b1/1, Product1/2, [Q]  "Power"
  b2/1 -> Out1/1
  [T] -> b2/1  "T"
  [Q] -> b2/2  "Q_kW"
  Source1/1 -> [T]
  Constant1/1 -> Switch1/3
  Product/1 -> Switch1/1  "Power"
  [Q] -> b1/2  "Q_kW"
  Gain/1 -> Sink1/1
